simulink model "CallJetSelect"  (R2017b)
settings: Solver=FixedStepAuto  StartTime=0.0  StopTime=10.0  FixedStep=0.08  RelTol=1e-3
model workspace (MAT data in the model file):
  ContractValidatorBlocksMap = containers.Map
  ContractValidatorBlocksMap.serialization.keys = {'CallJetSelect/ PRIMARY VERNIER Req/validator', 'CallJetSelect/contract/validator'}
  ContractValidatorBlocksMap.serialization.values{1}.block = 'CallJetSelect/ PRIMARY VERNIER Req/validator'
  ContractValidatorBlocksMap.serialization.values{1}.assumePorts = 0
  ContractValidatorBlocksMap.serialization.values{1}.guaranteePorts = 3
  ContractValidatorBlocksMap.serialization.values{1}.modeBlocksPorts = 0
  ContractValidatorBlocksMap.serialization.values{1}.portHandles.Inport = [3383.00195312 3384.0012207 3385.0012207]
  ContractValidatorBlocksMap.serialization.values{1}.portHandles.Outport = 3386.00134277
  ContractValidatorBlocksMap.serialization.values{1}.portHandles.Enable = []
  ContractValidatorBlocksMap.serialization.values{1}.portHandles.Trigger = []
  ContractValidatorBlocksMap.serialization.values{1}.portHandles.State = []
  ContractValidatorBlocksMap.serialization.values{1}.portHandles.LConn = []
  ContractValidatorBlocksMap.serialization.values{1}.portHandles.RConn = []
  ContractValidatorBlocksMap.serialization.values{1}.portHandles.Ifaction = []
  ContractValidatorBlocksMap.serialization.values{1}.portHandles.Reset = []
  ContractValidatorBlocksMap.serialization.values{1}.portConnectivity(1).Type = '1'
  ContractValidatorBlocksMap.serialization.values{1}.portConnectivity(1).Position = [365 -95]
  ContractValidatorBlocksMap.serialization.values{1}.portConnectivity(1).SrcBlock = 1916.00061035
  ContractValidatorBlocksMap.serialization.values{1}.portConnectivity(1).SrcPort = 0
  ContractValidatorBlocksMap.serialization.values{1}.portConnectivity(1).DstBlock = []
  ContractValidatorBlocksMap.serialization.values{1}.portConnectivity(1).DstPort = []
  ContractValidatorBlocksMap.serialization.values{1}.portConnectivity(2).Type = '2'
  ContractValidatorBlocksMap.serialization.values{1}.portConnectivity(2).Position = [365 75]
  ContractValidatorBlocksMap.serialization.values{1}.portConnectivity(2).SrcBlock = 1920.00134277
  ContractValidatorBlocksMap.serialization.values{1}.portConnectivity(2).SrcPort = 0
  ContractValidatorBlocksMap.serialization.values{1}.portConnectivity(2).DstBlock = []
  ContractValidatorBlocksMap.serialization.values{1}.portConnectivity(2).DstPort = []
  ContractValidatorBlocksMap.serialization.values{1}.portConnectivity(3).Type = '3'
  ContractValidatorBlocksMap.serialization.values{1}.portConnectivity(3).Position = [365 245]
  ContractValidatorBlocksMap.serialization.values{1}.portConnectivity(3).SrcBlock = 1924.00146484
  ContractValidatorBlocksMap.serialization.values{1}.portConnectivity(3).SrcPort = 0
  ContractValidatorBlocksMap.serialization.values{1}.portConnectivity(3).DstBlock = []
  ContractValidatorBlocksMap.serialization.values{1}.portConnectivity(3).DstPort = []
  ContractValidatorBlocksMap.serialization.values{1}.portConnectivity(4).Type = '1'
  ContractValidatorBlocksMap.serialization.values{1}.portConnectivity(4).Position = [500 75]
  ContractValidatorBlocksMap.serialization.values{1}.portConnectivity(4).SrcBlock = []
  ContractValidatorBlocksMap.serialization.values{1}.portConnectivity(4).SrcPort = []
  ContractValidatorBlocksMap.serialization.values{1}.portConnectivity(4).DstBlock = 1930.00146484
  ContractValidatorBlocksMap.serialization.values{1}.portConnectivity(4).DstPort = 0
  ContractValidatorBlocksMap.serialization.values{2}.block = 'CallJetSelect/contract/validator'
  ContractValidatorBlocksMap.serialization.values{2}.assumePorts = 1
  ContractValidatorBlocksMap.serialization.values{2}.guaranteePorts = 1
  ContractValidatorBlocksMap.serialization.values{2}.modeBlocksPorts = 3
  ContractValidatorBlocksMap.serialization.values{2}.portHandles.Inport = [10645.0003662 10644.0006104 10643.0003662 10642.0004883 10641.0004883]
  ContractValidatorBlocksMap.serialization.values{2}.portHandles.Outport = 10637.0004883
  ContractValidatorBlocksMap.serialization.values{2}.portHandles.Enable = []
  ContractValidatorBlocksMap.serialization.values{2}.portHandles.Trigger = []
  ContractValidatorBlocksMap.serialization.values{2}.portHandles.State = []
  ContractValidatorBlocksMap.serialization.values{2}.portHandles.LConn = []
  ContractValidatorBlocksMap.serialization.values{2}.portHandles.RConn = []
  ContractValidatorBlocksMap.serialization.values{2}.portHandles.Ifaction = []
  ContractValidatorBlocksMap.serialization.values{2}.portHandles.Reset = []
  ContractValidatorBlocksMap.serialization.values{2}.portConnectivity(1).Type = '1'
  ContractValidatorBlocksMap.serialization.values{2}.portConnectivity(1).Position = [365 -125]
  ContractValidatorBlocksMap.serialization.values{2}.portConnectivity(1).SrcBlock = 10661.0002441
  ContractValidatorBlocksMap.serialization.values{2}.portConnectivity(1).SrcPort = 0
  ContractValidatorBlocksMap.serialization.values{2}.portConnectivity(1).DstBlock = []
  ContractValidatorBlocksMap.serialization.values{2}.portConnectivity(1).DstPort = []
  ContractValidatorBlocksMap.serialization.values{2}.portConnectivity(2).Type = '2'
  ContractValidatorBlocksMap.serialization.values{2}.portConnectivity(2).Position = [365 -25]
  ContractValidatorBlocksMap.serialization.values{2}.portConnectivity(2).SrcBlock = 10665.0002441
  ContractValidatorBlocksMap.serialization.values{2}.portConnectivity(2).SrcPort = 0
  ContractValidatorBlocksMap.serialization.values{2}.portConnectivity(2).DstBlock = []
  ContractValidatorBlocksMap.serialization.values{2}.portConnectivity(2).DstPort = []
  ContractValidatorBlocksMap.serialization.values{2}.portConnectivity(3).Type = '3'
  ContractValidatorBlocksMap.serialization.values{2}.portConnectivity(3).Position = [365 75]
  ContractValidatorBlocksMap.serialization.values{2}.portConnectivity(3).SrcBlock = 10678.0003662
  ContractValidatorBlocksMap.serialization.values{2}.portConnectivity(3).SrcPort = 0
  ContractValidatorBlocksMap.serialization.values{2}.portConnectivity(3).DstBlock = []
  ContractValidatorBlocksMap.serialization.values{2}.portConnectivity(3).DstPort = []
  ContractValidatorBlocksMap.serialization.values{2}.portConnectivity(4).Type = '4'
  ContractValidatorBlocksMap.serialization.values{2}.portConnectivity(4).Position = [365 175]
  ContractValidatorBlocksMap.serialization.values{2}.portConnectivity(4).SrcBlock = 10703.0008545
  ContractValidatorBlocksMap.serialization.values{2}.portConnectivity(4).SrcPort = 0
  ContractValidatorBlocksMap.serialization.values{2}.portConnectivity(4).DstBlock = []
  ContractValidatorBlocksMap.serialization.values{2}.portConnectivity(4).DstPort = []
  ContractValidatorBlocksMap.serialization.values{2}.portConnectivity(5).Type = '5'
  ContractValidatorBlocksMap.serialization.values{2}.portConnectivity(5).Position = [365 275]
  ContractValidatorBlocksMap.serialization.values{2}.portConnectivity(5).SrcBlock = 10726.0004883
  ContractValidatorBlocksMap.serialization.values{2}.portConnectivity(5).SrcPort = 0
  ContractValidatorBlocksMap.serialization.values{2}.portConnectivity(5).DstBlock = []
  ContractValidatorBlocksMap.serialization.values{2}.portConnectivity(5).DstPort = []
  ContractValidatorBlocksMap.serialization.values{2}.portConnectivity(6).Type = '1'
  ContractValidatorBlocksMap.serialization.values{2}.portConnectivity(6).Position = [500 75]
  ContractValidatorBlocksMap.serialization.values{2}.portConnectivity(6).SrcBlock = []
  ContractValidatorBlocksMap.serialization.values{2}.portConnectivity(6).SrcPort = []
  ContractValidatorBlocksMap.serialization.values{2}.portConnectivity(6).DstBlock = 10587.0004883
  ContractValidatorBlocksMap.serialization.values{2}.portConnectivity(6).DstPort = 0
  ContractValidatorBlocksMap.serialization.uniformity = 0
  ContractValidatorBlocksMap.serialization.keyType = 'char'
  ContractValidatorBlocksMap.serialization.valueType = 'any'
undefined symbols (not defined in the file or in its folder): sldvsubsys
libraries: sldvlib x5, MATLAB_Function_lib x1
settings Model: Creator=hbourbou  LastModifiedBy=hbourbou

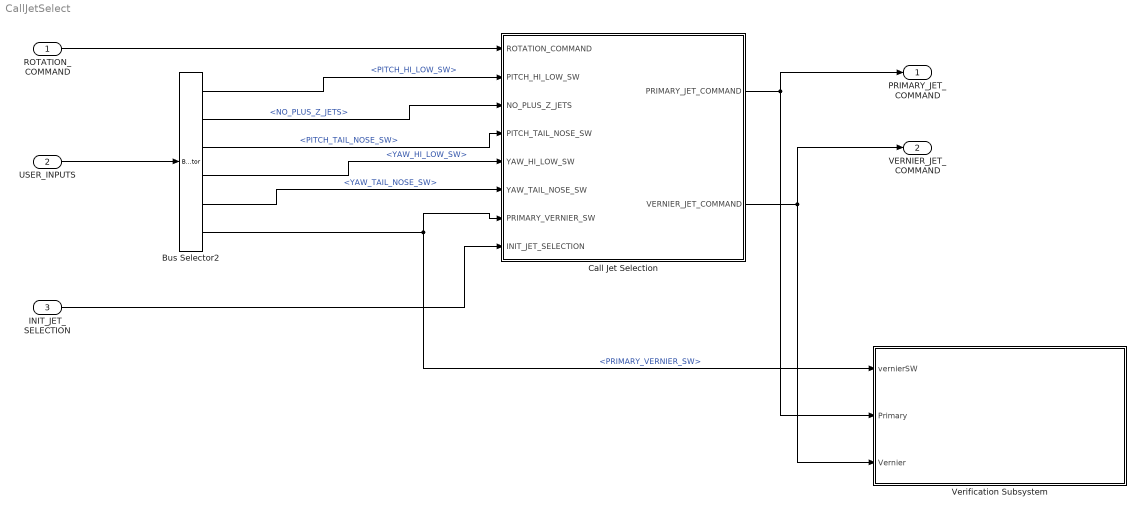
== system CallJetSelect ==
  ROTATION_COMMAND : Inport
  USER_INPUTS : Inport  Port=2  OutDataTypeStr=Bus: user_inputsBus
  INIT_JET_SELECTION : Inport  Port=3  OutDataTypeStr=boolean
  Bus Selector2 : BusSelector  OutputSignals=PITCH_HI_LOW_SW,NO_PLUS_Z_JETS,PITCH_TAIL_NOSE_SW,YAW_HI_LOW_SW,YAW_TAIL_NOSE_SW,PRIMARY_VERNIER_SW
  Call Jet Selection : Subsystem
  Verification Subsystem : Subsystem  Tag=VerificationSubsystem  DisableCoverage=on  LoadFcn=sldvsubsys('check')  TreatAsAtomicUnit=on  SimViewingDevice=on  mask(VerificationSubsystem){}
      mask init:
      | sldvsubsys('maskInit');
      settings: CopyFcn=sldvsubsys('copy');  OpenFcn=open_system(gcb,'force');
      settings: PreSaveFcn=|
      | set_param(gcb,'SimViewingDevice','on');
      | sldvsubsys('check');
      mask Help: helpview(fullfile(docroot,'toolbox','sldv','sldv.map'),'verificationsubsystem')
      mask Display: image(imread('sldvicon_versubsys.png','BackGroundColor',[1 1 1]),'center');
  PRIMARY_JET_COMMAND : Outport  OutDataTypeStr=boolean  PortDimensions=11
  VERNIER_JET_COMMAND : Outport  Port=2  OutDataTypeStr=boolean  PortDimensions=6
  wires:
  ROTATION_COMMAND/1 -> Call Jet Selection/1(ROTATION_COMMAND)
  Bus Selector2/1 -> Call Jet Selection/2(PITCH_HI_LOW_SW)  "<PITCH_HI_LOW_SW>"
  Bus Selector2/2 -> Call Jet Selection/3(NO_PLUS_Z_JETS)  "<NO_PLUS_Z_JETS>"
  Bus Selector2/3 -> Call Jet Selection/4(PITCH_TAIL_NOSE_SW)  "<PITCH_TAIL_NOSE_SW>"
  Bus Selector2/4 -> Call Jet Selection/5(YAW_HI_LOW_SW)  "<YAW_HI_LOW_SW>"
  Bus Selector2/5 -> Call Jet Selection/6(YAW_TAIL_NOSE_SW)  "<YAW_TAIL_NOSE_SW>"
  Bus Selector2/6 -> Verification Subsystem/1(vernierSW), Call Jet Selection/7(PRIMARY_VERNIER_SW)  "<PRIMARY_VERNIER_SW>"
  Call Jet Selection/2(VERNIER_JET_COMMAND) -> VERNIER_JET_COMMAND/1, Verification Subsystem/3(Vernier)
  Call Jet Selection/1(PRIMARY_JET_COMMAND) -> PRIMARY_JET_COMMAND/1, Verification Subsystem/2(Primary)
  USER_INPUTS/1 -> Bus Selector2/1
  INIT_JET_SELECTION/1 -> Call Jet Selection/8(INIT_JET_SELECTION)

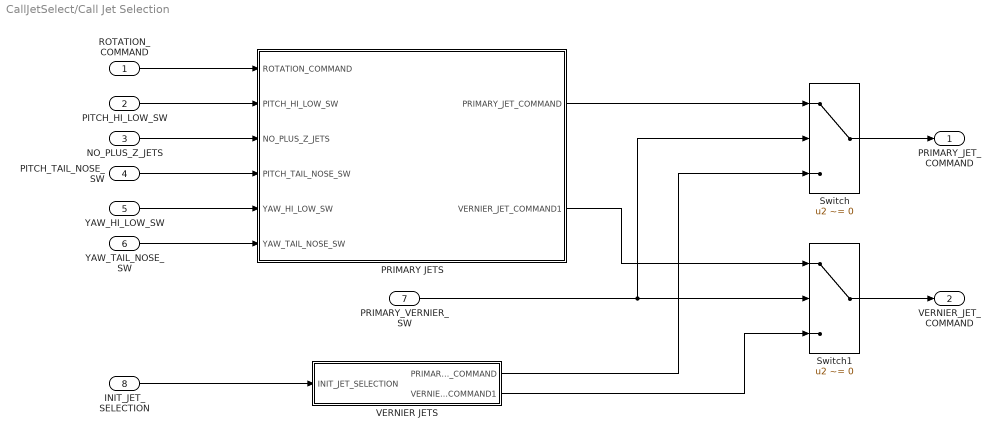
== system CallJetSelect/Call Jet Selection ==
  ROTATION_COMMAND : Inport
  PITCH_HI_LOW_SW : Inport  Port=2
  NO_PLUS_Z_JETS : Inport  Port=3
  PITCH_TAIL_NOSE_SW : Inport  Port=4
  YAW_HI_LOW_SW : Inport  Port=5
  YAW_TAIL_NOSE_SW : Inport  Port=6
  PRIMARY_VERNIER_SW : Inport  Port=7  OutDataTypeStr=boolean
  INIT_JET_SELECTION : Inport  Port=8
  PRIMARY JETS : Subsystem  TreatAsAtomicUnit=on
  Switch : Switch  Criteria=u2 ~= 0
  Switch1 : Switch  Criteria=u2 ~= 0
  VERNIER JETS : Subsystem  TreatAsAtomicUnit=on
  PRIMARY_JET_COMMAND : Outport  OutDataTypeStr=boolean  PortDimensions=11
  VERNIER_JET_COMMAND : Outport  Port=2  OutDataTypeStr=boolean  PortDimensions=6
  wires:
  NO_PLUS_Z_JETS/1 -> PRIMARY JETS/3(NO_PLUS_Z_JETS)
  PRIMARY JETS/1(PRIMARY_JET_COMMAND) -> Switch/1
  PITCH_HI_LOW_SW/1 -> PRIMARY JETS/2(PITCH_HI_LOW_SW)
  Switch/1 -> PRIMARY_JET_COMMAND/1
  VERNIER JETS/1(PRIMARY_JET_COMMAND) -> Switch/3
  ROTATION_COMMAND/1 -> PRIMARY JETS/1(ROTATION_COMMAND)
  VERNIER JETS/2(VERNIER_JET_COMMAND1) -> Switch1/3
  YAW_HI_LOW_SW/1 -> PRIMARY JETS/5(YAW_HI_LOW_SW)
  PITCH_TAIL_NOSE_SW/1 -> PRIMARY JETS/4(PITCH_TAIL_NOSE_SW)
  PRIMARY JETS/2(VERNIER_JET_COMMAND1) -> Switch1/1
  Switch1/1 -> VERNIER_JET_COMMAND/1
  YAW_TAIL_NOSE_SW/1 -> PRIMARY JETS/6(YAW_TAIL_NOSE_SW)
  PRIMARY_VERNIER_SW/1 -> Switch/2, Switch1/2
  INIT_JET_SELECTION/1 -> VERNIER JETS/1(INIT_JET_SELECTION)

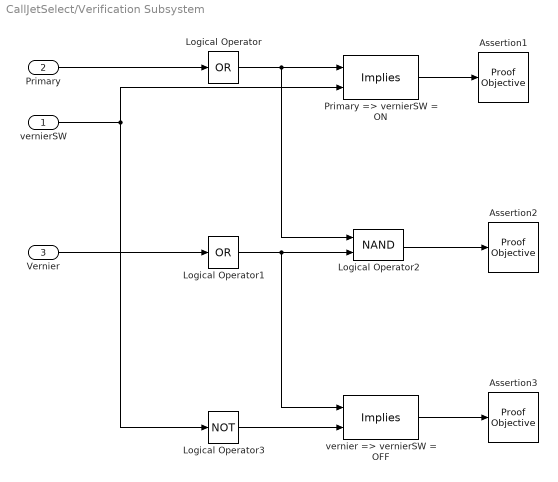
== system CallJetSelect/Verification Subsystem ==
  vernierSW : Inport
  Primary : Inport  Port=2
  Vernier : Inport  Port=3
  Assertion1 : sldvlib/Objectives and Constraints/Proof Objective  enabled=on  customAVTBlockType=Proof Objective  intervals=true  dispValues=on  outEnabled=off  enableStopSim=off
      settings: AttributesFormatString=%<intervals>  SourceProductName=Simulink Design Verifier  SourceProductBaseCode=DV
  Assertion2 : sldvlib/Objectives and Constraints/Proof Objective  enabled=on  customAVTBlockType=Proof Objective  intervals=true  dispValues=on  outEnabled=off  enableStopSim=off
      settings: AttributesFormatString=%<intervals>  SourceProductName=Simulink Design Verifier  SourceProductBaseCode=DV
  Assertion3 : sldvlib/Objectives and Constraints/Proof Objective  enabled=on  customAVTBlockType=Proof Objective  intervals=true  dispValues=on  outEnabled=off  enableStopSim=off
      settings: AttributesFormatString=%<intervals>  SourceProductName=Simulink Design Verifier  SourceProductBaseCode=DV
  Logical Operator : Logic  Operator=OR  Inputs=1  AllPortsSameDT=off  OutDataTypeStr=boolean
  Logical Operator1 : Logic  Operator=OR  Inputs=1  AllPortsSameDT=off  OutDataTypeStr=boolean
  Logical Operator2 : Logic  Operator=NAND  AllPortsSameDT=off  OutDataTypeStr=boolean
  Logical Operator3 : Logic  Operator=NOT  Inputs=1  AllPortsSameDT=off  OutDataTypeStr=boolean
  Primary => vernierSW = ON : sldvlib/Verification Utilities/Implies
      settings: SourceProductName=Simulink Design Verifier  SourceProductBaseCode=DV
  vernier => vernierSW = OFF : sldvlib/Verification Utilities/Implies
      settings: SourceProductName=Simulink Design Verifier  SourceProductBaseCode=DV
  wires:
  Vernier/1 -> Logical Operator1/1
  Logical Operator3/1 -> vernier => vernierSW = OFF/2
  Logical Operator/1 -> Logical Operator2/1, Primary => vernierSW = ON/1
  Primary/1 -> Logical Operator/1
  vernierSW/1 -> Primary => vernierSW = ON/2, Logical Operator3/1
  Logical Operator1/1 -> Logical Operator2/2, vernier => vernierSW = OFF/1
  Primary => vernierSW = ON/1 -> Assertion1/1
  Logical Operator2/1 -> Assertion2/1
  vernier => vernierSW = OFF/1 -> Assertion3/1

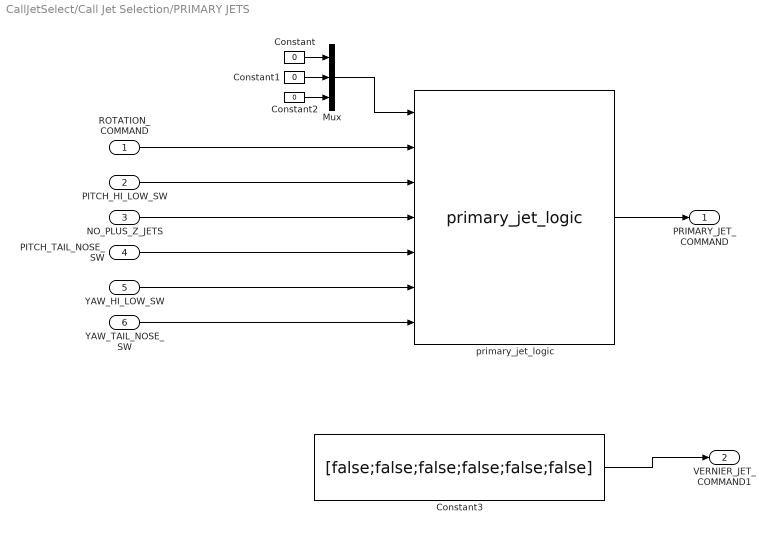
== system CallJetSelect/Call Jet Selection/PRIMARY JETS ==
  ROTATION_COMMAND : Inport
  PITCH_HI_LOW_SW : Inport  Port=2
  NO_PLUS_Z_JETS : Inport  Port=3
  PITCH_TAIL_NOSE_SW : Inport  Port=4
  YAW_HI_LOW_SW : Inport  Port=5
  YAW_TAIL_NOSE_SW : Inport  Port=6
  Constant : Constant  Value=0
  Constant1 : Constant  Value=0
  Constant2 : Constant  Value=0
  Constant3 : Constant  Value=[false;false;false;false;false;false]  OutDataTypeStr=boolean
  Mux : Mux  Inputs=3
  primary_jet_logic : MATLAB_Function_lib/primary_jet_logic
  PRIMARY_JET_COMMAND : Outport
  VERNIER_JET_COMMAND1 : Outport  Port=2
  wires:
  PITCH_TAIL_NOSE_SW/1 -> primary_jet_logic/5
  Mux/1 -> primary_jet_logic/1
  YAW_HI_LOW_SW/1 -> primary_jet_logic/6
  YAW_TAIL_NOSE_SW/1 -> primary_jet_logic/7
  NO_PLUS_Z_JETS/1 -> primary_jet_logic/4
  ROTATION_COMMAND/1 -> primary_jet_logic/2
  primary_jet_logic/1 -> PRIMARY_JET_COMMAND/1
  Constant2/1 -> Mux/3
  PITCH_HI_LOW_SW/1 -> primary_jet_logic/3
  Constant1/1 -> Mux/2
  Constant/1 -> Mux/1
  Constant3/1 -> VERNIER_JET_COMMAND1/1

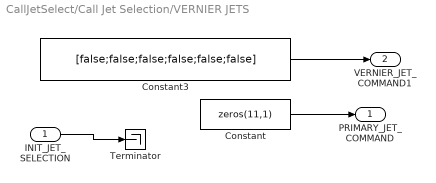
== system CallJetSelect/Call Jet Selection/VERNIER JETS ==
  INIT_JET_SELECTION : Inport
  Constant : Constant  Value=zeros(11,1)  VectorParams1D=off  OutDataTypeStr=boolean
  Constant3 : Constant  Value=[false;false;false;false;false;false]  OutDataTypeStr=boolean
  Terminator : Terminator
  PRIMARY_JET_COMMAND : Outport
  VERNIER_JET_COMMAND1 : Outport  Port=2
  wires:
  Constant/1 -> PRIMARY_JET_COMMAND/1
  Constant3/1 -> VERNIER_JET_COMMAND1/1
  INIT_JET_SELECTION/1 -> Terminator/1
